simulink model "mwrc04_fullvehicle"  (Simulink 6.0)
settings: Solver=ode3  SolverMode=SingleTasking  StartTime=0.0  StopTime=2  FixedStep=0.001  RelTol=1e-5  AbsTol=1e-6
PreLoadFcn:
  | load fsysdat
undefined symbols (not defined in the file or in its folder): A1, A2, B1, B2, converter_data, DISABLED, downtab, emap, hys, Iei, Ki, LOW, LSB, max_ego, max_press, max_speed, max_throt, min_press, min_throt, Neng_max, o2_t_thresh, Pbar, PressEst, pumpCon, RICH, sigbuilder_block, SpeedEst, ThrotEst, uptab, vehicledata, zero_thresh
libraries: simulink_extras x2, simulink x1
settings Model: Creator=nikita  LastModifiedBy=mshakeri  ExtModeTrigMode=oneshot  ExtModeArmWhenConnect=off  ExtModeAutoUpdateStatusClock=off  ProdHWDeviceType=Specified
settings SolverCC: AutoInsertRateTranBlk=on
settings DataIOCC: LimitDataPoints=off  SignalLoggingName=sigsOut
settings OptimizationCC: MultiInstanced=off
settings FormatCC: IgnoreBidirectionalLines=off
settings DebuggingCC: IntegerOverflowMsg=none
settings HardwareCC: ProdHWDeviceType=Specified
settings RTWCC: SystemTargetFile=ert.tlc  TemplateMakefile=ert_default_tmf  Description=RTW Embedded Coder  ProcessScript=ert_make_rtw_hook
settings CodeAppCC: IgnoreCustomStorageClasses=off  SimulinkBlockComments=off
settings ERTTargetCC: TargetFcnLib=iso_c_tmw.mat  GenerateSampleERTMain=on  GenFloatMathFcnCalls=ANSI_C  RootIOFormat=Individual Arguments  LifeSpan=1  SourceCodeTemplate=example_banner.tlc  HeaderCodeTemplate=example_banner.tlc  SourceDataTemplate=example_banner.tlc  HeaderDataTemplate=example_banner.tlc  ERTCustomFileTemplate=example_file_process.tlc  InitialValueSource=Model

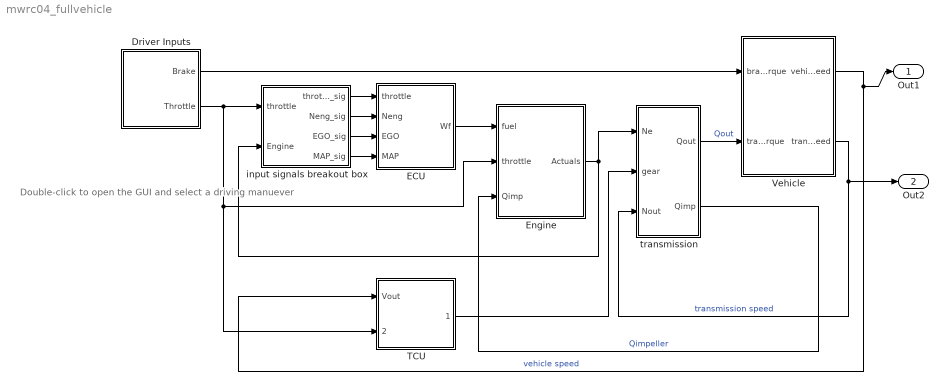
== system mwrc04_fullvehicle ==
  note: Double-click to
      | open the GUI
      | and select a
      | driving manuever
  Driver Inputs : Subsystem  Tag=STV Subsys  StartFcn=sigbuilder_block('start');  StopFcn=sigbuilder_block('stop');  ClipboardFcn=sigbuilder_block('clipboard');  mask(Sigbuilder block){}
      mask help: Sigbuilder GUI
      mask init:
      | tuvar = sigbuilder_block('maskInit');
      settings: CopyFcn=sigbuilder_block('copy');  DeleteFcn=sigbuilder_block('delete');  ModelCloseFcn=sigbuilder_block('modelClose');  PreSaveFcn=sigbuilder_block('preSave');  NameChangeFcn=sigbuilder_block('namechange');  OpenFcn=sigbuilder_block('open',[12 234.75 413.25 257.25 ]);  CloseFcn=sigbuilder_block('close');
      mask Display: plot(0,0,100,100,[10,10,40,40,10],[80,20,20,80,80],[40,10],[50,50], [40,27,10],[65,72,56],[40,25,25,10],[28,28,43,43]);
  ECU : Subsystem  TreatAsAtomicUnit=on
  Engine : Subsystem
  TCU : Subsystem  TreatAsAtomicUnit=on
  Vehicle : Subsystem  mask(vehicle model){Rfd=vehicledata(1), rload0=vehicledata(2), rload2=vehicledata(3), Rw=vehicledata(4), Iv=vehicledata(5), N20=vehicledata(6)/vehicledata(4)*vehicledata(1)}
      mask prompts: Rfd "final drive ratio"; rload0 "drag friction at wheels"; rload2 "aerodynamic drag"; Rw "wheel radius"; Iv "vehicle inertia"; N20 "initial transmission output speed"
      mask help: vehicle dynamics: torque input from trans., outputs are input speed (transmission output) and vehicle speed
      mask Display:
      | port_label('input',1,'Qbrake')
      | port_label('input',2,'Qtrans')
      | port_label('output',1,'Vout')
      | port_label('output',2,'Nout')
  input signals breakout box : Subsystem
  transmission : Subsystem
  Out1 : Outport
  Out2 : Outport  Port=2
  wires:
  ECU/1("Wf ") -> Engine/1(fuel)
  transmission/1(Qout) -> Vehicle/2(transmission output torque)  "Qout"
  Vehicle/1(vehicle speed) -> TCU/1(Vout), Out1/1  "vehicle speed"
  Driver Inputs/1(Brake) -> Vehicle/1(brake torque)
  input signals breakout box/1(throttle_sig) -> ECU/1(throttle)
  input signals breakout box/2(Neng_sig) -> ECU/2(Neng)
  input signals breakout box/3(EGO_sig) -> ECU/3(EGO)
  input signals breakout box/4(MAP_sig) -> ECU/4(MAP)
  TCU/1(gear select) -> transmission/2(gear)
  transmission/2(Qimp) -> Engine/3(Qimp)  "Qimpeller"
  Driver Inputs/2(Throttle) -> Engine/2(throttle), TCU/2(throttle), input signals breakout box/1(throttle)
  Engine/1(Actuals) -> transmission/1(Ne), input signals breakout box/2(Engine)
  Vehicle/2(transmission output speed) -> transmission/3(Nout), Out2/1  "transmission speed"

== system mwrc04_fullvehicle/Driver Inputs ==
  Demux : Demux  Tag=STV Demux  Outputs=2
  FromWs : FromWorkspace  Tag=STV FromWs  VariableName=tuvar  SampleTime=0.001  SigBuilderData=DataTag0
      SigBuilderData=|
      | channels(1).label = 'Brake'
      | channels(1).allXData = {[0 50], [0 50], [0 10 10 50], [0 50]}
      | channels(1).allYData = {[0 0], [0 0], [0 0 325 325], [0 0]}
      | channels(2).label = 'Throttle'
      | channels(2).allXData = {[0 14.9 15 15 50], [0 50], [0 5.1 5.1 50], [0 4.8 4.8 50]}
      | channels(2).allYData = {[60 40 100 100 58.8235294118], [13.4 24], [50 50 1 1], [80 80 1 1]}
      | dataSet(1).timeRange = [0 50]
      | dataSet(1).name = 'Passing Maneuver'
      | dataSet(2).timeRange = [0 50]
      | dataSet(2).name = 'Gradual Acceleration'
      | dataSet(3).timeRange = [0 50]
      | dataSet(3).name = 'Hard braking'
      | dataSet(4).timeRange = [0 50]
      | dataSet(4).name = 'Coasting'
  Brake : Outport  Tag=STV Outport
  Throttle : Outport  Tag=STV Outport  Port=2
  wires:
  FromWs/1 -> Demux/1
  Demux/1 -> Brake/1
  Demux/2 -> Throttle/1

== system mwrc04_fullvehicle/ECU ==
  note: Fuel Rate Control
  note: Physical Inputs
  note: Physical Outputs
  throttle : Inport
  Neng : Inport  Port=2
  EGO : Inport  Port=3
  MAP : Inport  Port=4
  Analog conditioning and conversion : Subsystem
  Analog output conversion : Subsystem
  ECU Application Software : Subsystem  TreatAsAtomicUnit=on
  "Wf " : Outport  InitialOutput=0
  wires:
  ECU Application Software/1(cmdOut) -> Analog output conversion/1(cmdOut)
  throttle/1 -> Analog conditioning and conversion/1(throttle_sig)  "throttle"
  Neng/1 -> Analog conditioning and conversion/2(Neng_sig)  "Neng"
  EGO/1 -> Analog conditioning and conversion/3(EGO_sig)  "EGO"
  MAP/1 -> Analog conditioning and conversion/4(MAP_sig)  "MAP"
  Analog conditioning and conversion/1(senseRaw) -> ECU Application Software/1(senseIn)
  Analog output conversion/1(Wf) -> "Wf "/1

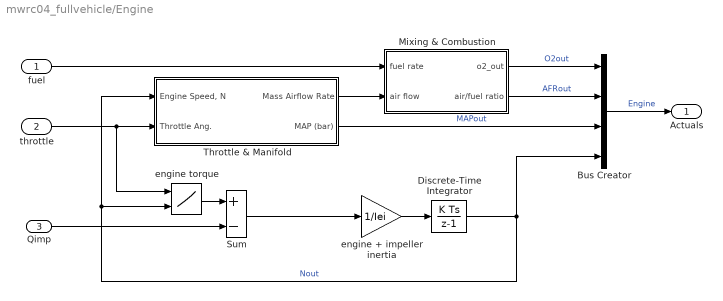
== system mwrc04_fullvehicle/Engine ==
  fuel : Inport
  throttle : Inport  Port=2
  Qimp : Inport  Port=3
  Bus Creator : BusCreator
  Discrete-Time Integrator : DiscreteIntegrator  InitialCondition=1000  LimitOutput=on  UpperSaturationLimit=Neng_max  LowerSaturationLimit=600  SampleTime=0.001
  Mixing & Combustion : Subsystem
  Sum : Sum  Inputs=+-  SaturateOnIntegerOverflow=on  InputSameDT=on
  Throttle & Manifold : Subsystem
  engine torque : Lookup2D  RowIndex=thvec  ColumnIndex=nevec  OutputValues=emap  OutScaling=2^-10  InputSameDT=on
  engine + impeller inertia : Gain  Gain=1/Iei  SaturateOnIntegerOverflow=on
  Actuals : Outport
  wires:
  Throttle & Manifold/1(Mass Airflow Rate) -> Mixing & Combustion/2(air flow)
  fuel/1 -> Mixing & Combustion/1(fuel rate)
  throttle/1 -> Throttle & Manifold/2(Throttle Ang.), engine torque/1
  Mixing & Combustion/2(air/fuel ratio) -> Bus Creator/2  "AFRout"
  Throttle & Manifold/2(MAP (bar)) -> Bus Creator/3  "MAPout"
  Mixing & Combustion/1(o2_out) -> Bus Creator/1  "O2out"
  Bus Creator/1 -> Actuals/1  "Engine"
  Discrete-Time Integrator/1 -> engine torque/2, Throttle & Manifold/1("Engine Speed, N"), Bus Creator/4  "Nout"
  Sum/1 -> engine + impeller inertia/1
  engine + impeller inertia/1 -> Discrete-Time Integrator/1
  engine torque/1 -> Sum/1
  Qimp/1 -> Sum/2

== system mwrc04_fullvehicle/TCU ==
  note: Electronic Shift Control
  Vout : Inport
  throttle : Inport  Port=2
  Threshold Calculation : Subsystem  Orientation=left  TreatAsAtomicUnit=on
  shift_logic : Stateflow chart
  gear select : Outport
  wires:
  Threshold Calculation/1(down_th) -> shift_logic/3(down_th)
  Threshold Calculation/2(up_th) -> shift_logic/2(up_th)
  shift_logic/1(gear) -> Threshold Calculation/1(gear), gear select/1
  shift_logic/2(CALC_TH) -> Threshold Calculation/Trigger
  throttle/1 -> Threshold Calculation/2(throttle)
  Vout/1 -> shift_logic/1(speed)

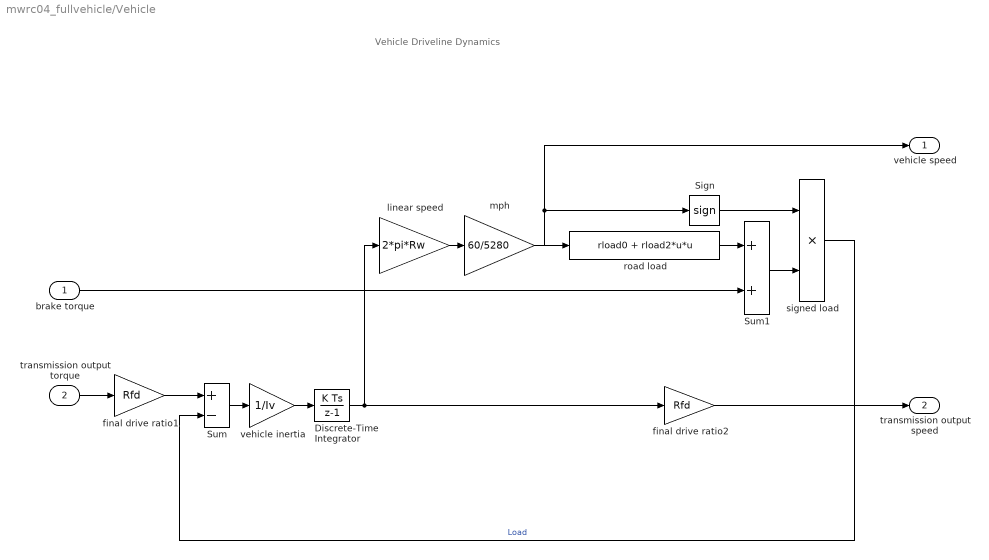
== system mwrc04_fullvehicle/Vehicle ==
  note: Vehicle Driveline Dynamics
  brake torque : Inport
  transmission output torque : Inport  Port=2
  Discrete-Time Integrator : DiscreteIntegrator  InitialCondition=N20/Rfd  SampleTime=0.001
  Sign : Signum
  Sum : Sum  Inputs=+-  SaturateOnIntegerOverflow=on  InputSameDT=on
  Sum1 : Sum  SaturateOnIntegerOverflow=on  InputSameDT=on
  final drive ratio1 : Gain  Gain=Rfd  SaturateOnIntegerOverflow=on
  final drive ratio2 : Gain  Gain=Rfd  SaturateOnIntegerOverflow=on
  linear speed : Gain  Gain=2*pi*Rw  SaturateOnIntegerOverflow=on
  mph : Gain  Gain=60/5280  SaturateOnIntegerOverflow=on
  road load : Fcn  Expr=rload0 + rload2*u*u
  signed load : Product  SaturateOnIntegerOverflow=on  InputSameDT=on
  vehicle inertia : Gain  Gain=1/Iv  SaturateOnIntegerOverflow=on
  vehicle speed : Outport  InitialOutput=0
  transmission output speed : Outport  Port=2  InitialOutput=0
  wires:
  final drive ratio2/1 -> transmission output speed/1
  brake torque/1 -> Sum1/2
  Sum1/1 -> signed load/2
  road load/1 -> Sum1/1
  Sign/1 -> signed load/1
  signed load/1 -> Sum/2  "Load"
  transmission output torque/1 -> final drive ratio1/1
  vehicle inertia/1 -> Discrete-Time Integrator/1
  Sum/1 -> vehicle inertia/1
  mph/1 -> vehicle speed/1, Sign/1, road load/1
  linear speed/1 -> mph/1
  Discrete-Time Integrator/1 -> final drive ratio2/1, linear speed/1
  final drive ratio1/1 -> Sum/1

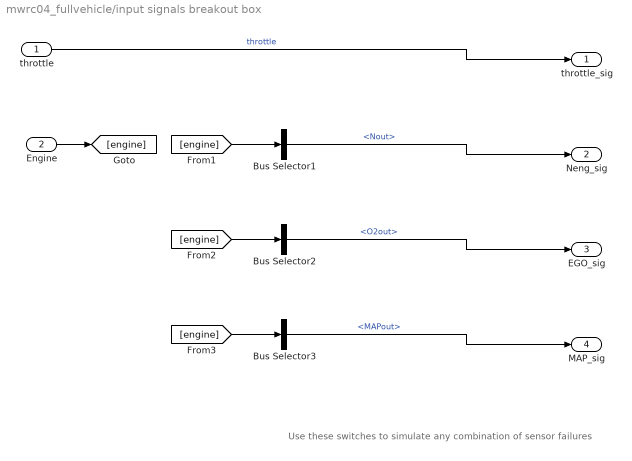
== system mwrc04_fullvehicle/input signals breakout box ==
  note: Use these switches to
      | simulate any combination
      | of sensor failures
  throttle : Inport
  Engine : Inport  Port=2
  Bus Selector1 : BusSelector  OutputSignals=Nout
  Bus Selector2 : BusSelector  OutputSignals=O2out
  Bus Selector3 : BusSelector  OutputSignals=MAPout
  throttle_sig : Outport
  Neng_sig : Outport  Port=2
  EGO_sig : Outport  Port=3
  MAP_sig : Outport  Port=4
  wires:
  throttle/1 -> throttle_sig/1  "throttle"
  Bus Selector2/1 -> EGO_sig/1  "<O2out>"
  Bus Selector3/1 -> MAP_sig/1  "<MAPout>"
  Bus Selector1/1 -> Neng_sig/1  "<Nout>"
  Engine/1 -> [engine]
  [engine] -> Bus Selector1/1
  [engine] -> Bus Selector2/1
  [engine] -> Bus Selector3/1

== system mwrc04_fullvehicle/transmission ==
  Ne : Inport
  gear : Inport  Port=2
  Nout : Inport  Port=3
  Bus Selector1 : BusSelector  OutputSignals=Nout
  Torque Converter : Subsystem  mask(torque converter){speedratio=converter_data(:,1), Kfactor=converter_data(:,2), Torkratio=converter_data(:,3)}
      mask prompts: speedratio "speed ratio"; Kfactor "K factor"; Torkratio "torque ratio"
      mask help: torque converter
      mask Help: Torque converter input and output torques are computed as a function of the input and output speeds
      mask Display: plot([cos([90:10:450]*pi/180),.63*cos([90:10:450]*pi/180),.63*cos([90:10:240]*pi/180),cos([240:10:300]*pi/180),.63*cos([300]*pi/180)],[sin([90:10:450]*pi/180),.63*sin([90:10:450]*pi/180)+.1,.63*sin([90:10:240]*pi/180)+.1,sin([240:10:300]*pi/180),.63*sin([300]*pi/180)+.1])
  transmission ratio : Subsystem
  Qout : Outport  InitialOutput=0
  Qimp : Outport  Port=2  InitialOutput=0
  wires:
  transmission ratio/1(Tout) -> Qout/1
  Torque Converter/1(Ti) -> Qimp/1
  Nout/1 -> transmission ratio/3(Nout)
  gear/1 -> transmission ratio/2(gear)
  Ne/1 -> Bus Selector1/1
  transmission ratio/2(Nin) -> Torque Converter/2(Nin)
  Torque Converter/2(Tt) -> transmission ratio/1(Tin)  "turbine torque"
  Bus Selector1/1 -> Torque Converter/1(Neng)  "<Nout>"

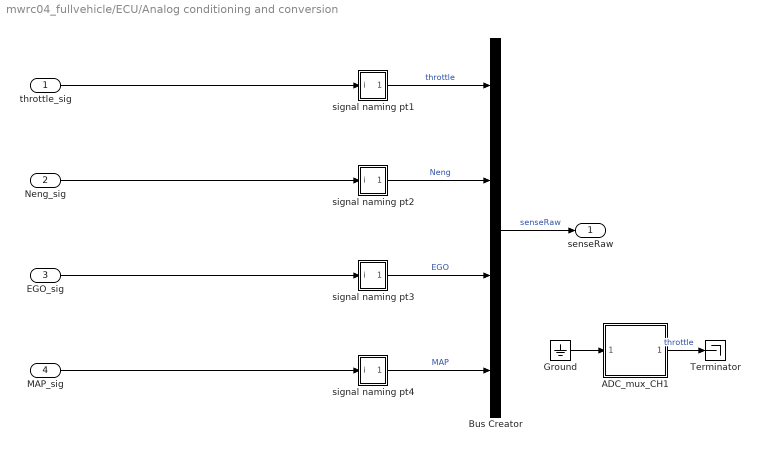
== system mwrc04_fullvehicle/ECU/Analog conditioning and conversion ==
  throttle_sig : Inport
  Neng_sig : Inport  Port=2
  EGO_sig : Inport  Port=3
  MAP_sig : Inport  Port=4
  ADC_mux_CH1 : Subsystem  mask(IdealADC){NumberOfConverterBits=8, Vmin=0, Vmax=5, OutputDataType=double}
      mask prompts: NumberOfConverterBits "Number of converter bits:"; Vmin "Min input voltage at low output:"; Vmax "Max input voltage at 2^n output (unreachable):"; OutputDataType "Output data type:"
      mask help: Idealized analog to digital converter. There are 2^n possible digital output codes for an n-bit converter. Each value represents an equal fraction of the total analog input range in steps of one least significant bit (1 LSB). 1 LSB is (Vmax - Vmin)/2^bits. The midpoint of these steps corresponds to the actual value and thus introduce quantization error that is never more than 1/2 LSB. Since the first and last steps in the converter's range are only 1/2 LSB in width, the full scale range (FSR) of the converter is equal to (2^n - 1) step widths. The FSR low transition occurs at Vmin + 1/2 LSB, the FSR high transition occurs at Vmax - 3/2 LSB. When the block output is a floating point type, int32 is used for truncation. Conversion time is zero in this model.
      mask init:
      | [LSB,steps_x,steps_y,line_xy] = sl_addamask(NumberOfConverterBits,Vmin,Vmax,OutputDataType);
      settings: AttributesFormatString=(settings: %<NumberOfConverterBits>-bit converter\nVmin: %<Vmin>, Vmax: %<Vmax>)
      mask Help: Use this block to model an ideal analog to digital converter.  To model non-ideal converters, it is suggested to use a direct look-up table to represent static errors and dynamic models for transient error sources.  Use a discrete delay of the appropriate duration to model conversion latency if this is a significant value in your application.  If there is an input mux, model this with triggered latencies on the input side of the A/D block.
      mask StyleString: edit,edit,edit,popup(double|single|int8|uint8|int16|uint16|int32|uint32|boolean)
      mask Display:
      | plot(steps_x,steps_y)
      | plot(line_xy, line_xy)
      | port_label('input',1,'A')
      | port_label('output',1,'D')
      | text(0.5,0.9,[num2str(NumberOfConverterBits),' bits'],'horizontalalignment','center')
  Bus Creator : BusCreator
  Ground : Ground
  Terminator : Terminator
  signal naming pt1 : Subsystem
  signal naming pt2 : Subsystem
  signal naming pt3 : Subsystem
  signal naming pt4 : Subsystem
  senseRaw : Outport
  wires:
  Bus Creator/1 -> senseRaw/1  "senseRaw"
  throttle_sig/1 -> signal naming pt1/1(i)
  Neng_sig/1 -> signal naming pt2/1(i)
  EGO_sig/1 -> signal naming pt3/1(i)
  MAP_sig/1 -> signal naming pt4/1(i)
  signal naming pt1/1(o) -> Bus Creator/1  "throttle"
  signal naming pt2/1(o) -> Bus Creator/2  "Neng"
  signal naming pt3/1(o) -> Bus Creator/3  "EGO"
  signal naming pt4/1(o) -> Bus Creator/4  "MAP"
  ADC_mux_CH1/1(Digital Counts) -> Terminator/1  "throttle"
  Ground/1 -> ADC_mux_CH1/1(Sampled Volts)

== system mwrc04_fullvehicle/ECU/Analog output conversion ==
  cmdOut : Inport
  Bus Selector : BusSelector  OutputSignals=Wfcmd
  signal naming pt1 : Subsystem
  Wf : Outport
  wires:
  cmdOut/1 -> Bus Selector/1
  Bus Selector/1 -> signal naming pt1/1(i)  "<Wfcmd>"
  signal naming pt1/1(o) -> Wf/1  "Wf"

== system mwrc04_fullvehicle/ECU/ECU Application Software ==
  note: ECU Application - Top Level
  senseIn : Inport
  Airflow calculation : Subsystem  TreatAsAtomicUnit=on
  Fuel  Calculation : Subsystem  TreatAsAtomicUnit=on
  Input Signal Conversion : Subsystem  TreatAsAtomicUnit=on
  Mode Logic : Subsystem  TreatAsAtomicUnit=on
  Output Signal Conversion : Subsystem  TreatAsAtomicUnit=on
  Sensor correction and  Fault Redundancy : Subsystem  TreatAsAtomicUnit=on
  cmdOut : Outport
  wires:
  Mode Logic/2(fuel_mode) -> Fuel  Calculation/4(mode), Airflow calculation/3(mode)
  Airflow calculation/2(feedback correction) -> Fuel  Calculation/2(feedback correction)
  Airflow calculation/1(est. air flow) -> Fuel  Calculation/1(est. air flow)
  Sensor correction and  Fault Redundancy/1(corrected) -> Airflow calculation/1(sens_in)
  Mode Logic/1(fail_state) -> Sensor correction and  Fault Redundancy/2(failures), Airflow calculation/2(Failures), Fuel  Calculation/3(Failures)
  senseIn/1 -> Input Signal Conversion/1(senseRaw)
  Fuel  Calculation/1(Cmd) -> Output Signal Conversion/1(Cmd)
  Output Signal Conversion/1(cmdOut) -> cmdOut/1
  Input Signal Conversion/1(sensors) -> Sensor correction and  Fault Redundancy/1(sensors), Mode Logic/1(sensors)

== system mwrc04_fullvehicle/Engine/Mixing & Combustion ==
  fuel rate : Inport
  air flow : Inport  Port=2
  Constant4 : Constant  Orientation=up  Value=0.1
  Discrete Transfer Fcn : DiscreteTransferFcn  Numerator=3  Denominator=[1 3]  SampleTime=0.001
  EGO Sensor : Fcn  Expr=(1-tanh(4*(u[1]-14.6)))/2
  MinMax : MinMax  Function=max  Inputs=2  SaturateOnIntegerOverflow=on  InputSameDT=on
  Product : Product  Inputs=*/  SaturateOnIntegerOverflow=on  InputSameDT=on
  o2_out : Outport  InitialOutput=0
  air/fuel ratio : Outport  Port=2  InitialOutput=0
  wires:
  Constant4/1 -> MinMax/2
  fuel rate/1 -> MinMax/1
  MinMax/1 -> Product/2
  Product/1 -> Discrete Transfer Fcn/1
  Discrete Transfer Fcn/1 -> air/fuel ratio/1, EGO Sensor/1
  EGO Sensor/1 -> o2_out/1
  air flow/1 -> Product/1

== system mwrc04_fullvehicle/Engine/Throttle & Manifold ==
  note: Air-Fuel Intake Dynamics
  "Engine Speed, N" : Inport
  Throttle Ang. : Inport  Port=2
  "Atmospheric Pressure, Pa (bar)" : Constant  Value=Pbar
  Intake Manifold : Subsystem
  Limit to Positive : Saturate  UpperLimit=inf  LowerLimit=0
  Throttle : Subsystem
  Mass Airflow Rate : Outport  InitialOutput=0
  MAP (bar) : Outport  Port=2  InitialOutput=0
  wires:
  Limit to Positive/1 -> Throttle/1("Throttle Angle, theta (deg)")
  Throttle Ang./1 -> Limit to Positive/1
  Throttle/1("Throttle  Flow, mdot  (g/s)") -> Intake Manifold/1(mdot Input  (g/s))
  "Engine Speed, N"/1 -> Intake Manifold/2(N (rad/sec))
  Intake Manifold/1(mdot to Cylinder  (g/s)) -> Mass Airflow Rate/1
  "Atmospheric Pressure, Pa (bar)"/1 -> Throttle/3("Atmospheric Pressure, Pa (bar) ")
  Intake Manifold/2("Manifold Pressure, Pm (bar)") -> Throttle/2("Manifold Pressure, Pm (bar)"), MAP (bar)/1

== system mwrc04_fullvehicle/TCU/Threshold Calculation ==
  gear : Inport
  throttle : Inport  Port=2
  run : TriggerPort  TriggerType=function-call  ZeroCross=off
  interp_down : Lookup2D  RowIndex=downth  ColumnIndex=[1:4]  OutputValues=downtab  OutScaling=2^-10  InputSameDT=on
  interp_up : Lookup2D  RowIndex=upth  ColumnIndex=[1:4]  OutputValues=uptab  OutScaling=2^-10  InputSameDT=on
  down_th : Outport
  up_th : Outport  Port=2
  wires:
  interp_up/1 -> up_th/1
  interp_down/1 -> down_th/1
  throttle/1 -> interp_up/1, interp_down/1
  gear/1 -> interp_up/2, interp_down/2

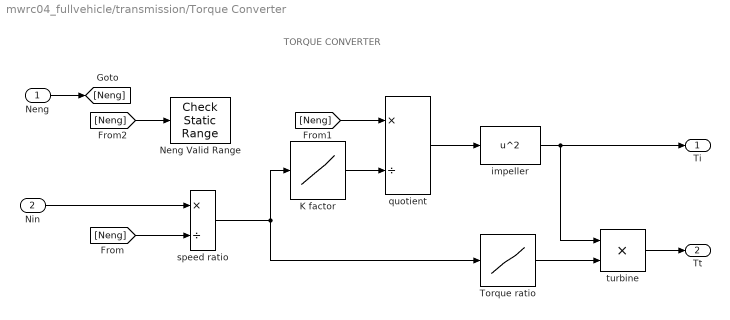
== system mwrc04_fullvehicle/transmission/Torque Converter ==
  note: TORQUE CONVERTER
  Neng : Inport
  Nin : Inport  Port=2
  K factor : Lookup  InputValues=speedratio  OutputValues=Kfactor  SaturateOnIntegerOverflow=on
  Neng Valid Range : simulink/Model Verification/Check  Static Range  Description=0 < u <= Neng_max  max=Neng_max  max_included=on  min=0  min_included=off  enabled=on  stopWhenAssertionFail=on  export=off  icon=graphic
      settings: AttributesFormatString=%<min> <= u <= %<max>
  Torque ratio : Lookup  InputValues=speedratio  OutputValues=Torkratio  SaturateOnIntegerOverflow=on
  impeller : Fcn  Expr=u^2
  quotient : Product  Inputs=*/  SaturateOnIntegerOverflow=on  InputSameDT=on
  speed ratio : Product  Inputs=*/  SaturateOnIntegerOverflow=on  InputSameDT=on
  turbine : Product  SaturateOnIntegerOverflow=on  InputSameDT=on
  Ti : Outport  InitialOutput=0
  Tt : Outport  Port=2  InitialOutput=0
  wires:
  quotient/1 -> impeller/1
  K factor/1 -> quotient/2
  impeller/1 -> Ti/1, turbine/1
  turbine/1 -> Tt/1
  Nin/1 -> speed ratio/1
  Torque ratio/1 -> turbine/2
  [Neng] -> speed ratio/2
  Neng/1 -> [Neng]
  [Neng] -> quotient/1
  [Neng] -> Neng Valid Range/1
  speed ratio/1 -> K factor/1, Torque ratio/1

== system mwrc04_fullvehicle/transmission/transmission ratio ==
  Tin : Inport
  gear : Inport  Port=2
  Nout : Inport  Orientation=left  Port=3
  Look-Up Table : Lookup  InputValues=[1 2 3 4]  OutputValues=[2.393 1.450 1.000 0.677]  SaturateOnIntegerOverflow=on
  Product : Product  SaturateOnIntegerOverflow=on  InputSameDT=on
  Product1 : Product  Orientation=left  SaturateOnIntegerOverflow=on  InputSameDT=on
  Tout : Outport  InitialOutput=0
  Nin : Outport  Orientation=left  Port=2  InitialOutput=0
  wires:
  Look-Up Table/1 -> Product1/1, Product/2
  Nout/1 -> Product1/2
  Product1/1 -> Nin/1
  Product/1 -> Tout/1
  Tin/1 -> Product/1
  gear/1 -> Look-Up Table/1

== system mwrc04_fullvehicle/ECU/Analog conditioning and conversion/ADC_mux_CH1 ==
  Sampled Volts : Inport
  ADC Counts Range divided by Input Voltage Range : Gain  Gain=1/LSB  SaturateOnIntegerOverflow=on
  Cause rounding behavior upon truncation : Constant  Orientation=up  Value=0.5
  Saturate voltage  to output range : Saturate  UpperLimit=Vmax - 1.5 * LSB  LowerLimit=Vmin + 0.5 * LSB
      settings: AttributesFormatString=Max = %<UpperLimit>\nMin = %<LowerLimit>
  Sum : Sum  Inputs=|++  SaturateOnIntegerOverflow=on
  cast : DataTypeConversion  OutDataTypeMode=double  RndMeth=Zero
  truncate : DataTypeConversion  OutDataTypeMode=int32  SaturateOnIntegerOverflow=on  RndMeth=Zero
  Digital Counts : Outport
  wires:
  Sampled Volts/1 -> Saturate voltage  to output range/1
  truncate/1 -> cast/1
  ADC Counts Range divided by Input Voltage Range/1 -> Sum/1
  Sum/1 -> truncate/1
  Cause rounding behavior upon truncation/1 -> Sum/2
  Saturate voltage  to output range/1 -> ADC Counts Range divided by Input Voltage Range/1
  cast/1 -> Digital Counts/1

== system mwrc04_fullvehicle/ECU/Analog conditioning and conversion/signal naming pt1 ==
  i : Inport
  o : Outport
  wires:
  i/1 -> o/1

== system mwrc04_fullvehicle/ECU/Analog conditioning and conversion/signal naming pt2 ==
  i : Inport
  o : Outport
  wires:
  i/1 -> o/1

== system mwrc04_fullvehicle/ECU/Analog conditioning and conversion/signal naming pt3 ==
  i : Inport
  o : Outport
  wires:
  i/1 -> o/1

== system mwrc04_fullvehicle/ECU/Analog conditioning and conversion/signal naming pt4 ==
  i : Inport
  o : Outport
  wires:
  i/1 -> o/1

== system mwrc04_fullvehicle/ECU/Analog output conversion/signal naming pt1 ==
  i : Inport
  o : Outport
  wires:
  i/1 -> o/1

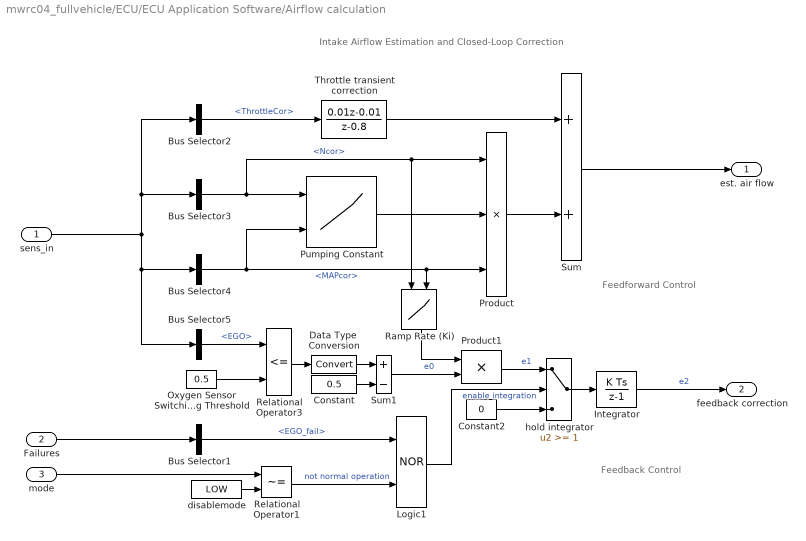
== system mwrc04_fullvehicle/ECU/ECU Application Software/Airflow calculation ==
  note: Intake Airflow Estimation and Closed-Loop Correction
  note: Feedback Control
  note: Feedforward Control
  sens_in : Inport
  Failures : Inport  Port=2
  mode : Inport  Port=3
  Bus Selector1 : BusSelector  OutputSignals=EGO_fail
  Bus Selector2 : BusSelector  OutputSignals=ThrottleCor
  Bus Selector3 : BusSelector  OutputSignals=Ncor
  Bus Selector4 : BusSelector  OutputSignals=MAPcor
  Bus Selector5 : BusSelector  OutputSignals=EGO
  Constant : Constant  Value=0.5
  Constant2 : Constant  Value=0
  Data Type  Conversion : DataTypeConversion  OutDataTypeMode=double  SaturateOnIntegerOverflow=on  RndMeth=Zero
  Integrator : DiscreteIntegrator  InitialCondition=-0.01  SampleTime=.01
  Logic1 : Logic  Operator=NOR
  Oxygen Sensor Switching Threshold : Constant  Value=0.5
  Product : Product  Inputs=3  SaturateOnIntegerOverflow=on  InputSameDT=on
  Product1 : Product  SaturateOnIntegerOverflow=on  InputSameDT=on
  Pumping Constant : Lookup2D  RowIndex=SpeedVect  ColumnIndex=press  OutputValues=pumpCon  SaturateOnIntegerOverflow=on  InputSameDT=on
  Ramp Rate (Ki) : Lookup2D  Orientation=down  RowIndex=[100:100:500]  ColumnIndex=[0:0.2:1]  OutputValues=[1:5]'*[1:6]*Ki  SaturateOnIntegerOverflow=on  InputSameDT=on
  Relational Operator1 : RelationalOperator  Operator=~=  InputSameDT=on
  Relational Operator3 : RelationalOperator  Operator=<=  InputSameDT=on
  Sum : Sum  Inputs=2  SaturateOnIntegerOverflow=on  InputSameDT=on
  Sum1 : Sum  Inputs=+-  SaturateOnIntegerOverflow=on  InputSameDT=on
  Throttle transient correction : DiscreteTransferFcn  Numerator=[0.01 -0.01]  Denominator=[1 -0.8]  SampleTime=.01
  disablemode : Constant  Value=LOW
  hold integrator : Switch  Threshold=1  SaturateOnIntegerOverflow=on  InputSameDT=on
  est. air flow : Outport  InitialOutput=0
  feedback correction : Outport  Port=2  InitialOutput=0
  wires:
  Integrator/1 -> feedback correction/1  "e2"
  mode/1 -> Relational Operator1/1
  sens_in/1 -> Bus Selector5/1, Bus Selector4/1, Bus Selector2/1, Bus Selector3/1
  Pumping Constant/1 -> Product/2
  Product/1 -> Sum/2
  Bus Selector4/1 -> Ramp Rate (Ki)/2, Product/3, Pumping Constant/2  "<MAPcor>"
  Bus Selector3/1 -> Pumping Constant/1, Product/1, Ramp Rate (Ki)/1  "<Ncor>"
  Throttle transient correction/1 -> Sum/1
  Sum/1 -> est. air flow/1
  Bus Selector2/1 -> Throttle transient correction/1  "<ThrottleCor>"
  Bus Selector1/1 -> Logic1/1  "<EGO_fail>"
  Failures/1 -> Bus Selector1/1
  disablemode/1 -> Relational Operator1/2
  Relational Operator1/1 -> Logic1/2  "not normal operation"
  Bus Selector5/1 -> Relational Operator3/1  "<EGO>"
  Oxygen Sensor Switching Threshold/1 -> Relational Operator3/2
  Ramp Rate (Ki)/1 -> Product1/1
  Constant2/1 -> hold integrator/3
  Product1/1 -> hold integrator/1  "e1"
  hold integrator/1 -> Integrator/1
  Logic1/1 -> hold integrator/2  "enable integration"
  Sum1/1 -> Product1/2  "e0"
  Relational Operator3/1 -> Data Type  Conversion/1
  Data Type  Conversion/1 -> Sum1/1
  Constant/1 -> Sum1/2

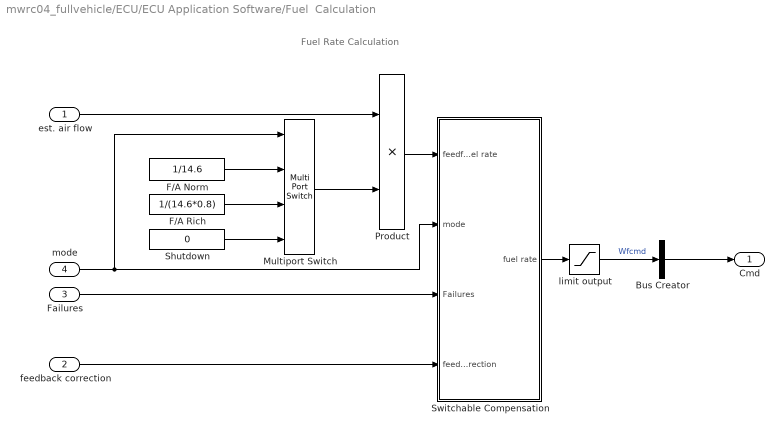
== system mwrc04_fullvehicle/ECU/ECU Application Software/Fuel  Calculation ==
  note: Fuel Rate Calculation
  est. air flow : Inport
  feedback correction : Inport  Port=2
  Failures : Inport  Port=3
  mode : Inport  Port=4
  Bus Creator : BusCreator  Inputs=1
  F/A Norm : Constant  Value=1/14.6
  F/A Rich : Constant  Value=1/(14.6*0.8)
  Multiport Switch : MultiPortSwitch  Inputs=3  SaturateOnIntegerOverflow=on  InputSameDT=on
  Product : Product  SaturateOnIntegerOverflow=on  InputSameDT=on
  Shutdown : Constant  Value=0
  Switchable Compensation : Subsystem
  limit output : Saturate  UpperLimit=100  LowerLimit=0
  Cmd : Outport  InitialOutput=0
  wires:
  limit output/1 -> Bus Creator/1  "Wfcmd"
  feedback correction/1 -> Switchable Compensation/4(feedback correction)
  Shutdown/1 -> Multiport Switch/4
  F/A Rich/1 -> Multiport Switch/3
  F/A Norm/1 -> Multiport Switch/2
  est. air flow/1 -> Product/1
  Multiport Switch/1 -> Product/2
  mode/1 -> Switchable Compensation/2(mode), Multiport Switch/1
  Failures/1 -> Switchable Compensation/3(Failures)
  Product/1 -> Switchable Compensation/1(feedforward fuel rate)
  Switchable Compensation/1(fuel rate) -> limit output/1
  Bus Creator/1 -> Cmd/1

== system mwrc04_fullvehicle/ECU/ECU Application Software/Input Signal Conversion ==
  note: Convert A/D counts to engineering units,
      | accounting for sensor nonlinearities
  senseRaw : Inport
  sensors : Outport
  wires:
  senseRaw/1 -> sensors/1

== system mwrc04_fullvehicle/ECU/ECU Application Software/Mode Logic ==
  sensors : Inport
  Bus Creator : BusCreator
  Bus Selector : BusSelector  OutputSignals=throttle,Neng,EGO,MAP
  Demux : Demux
  control logic : Stateflow chart  Description=Stateflow diagram to determine control system operating mode
  fail_state : Outport
  fuel_mode : Outport  Port=2
  wires:
  control logic/2(fuel_mode) -> fuel_mode/1
  sensors/1 -> Bus Selector/1
  Bus Selector/1 -> control logic/1(throt)  "<throttle>"
  Bus Selector/2 -> control logic/2(speed)  "<Neng>"
  Bus Selector/3 -> control logic/3(Ego)  "<EGO>"
  Bus Selector/4 -> control logic/4(press)  "<MAP>"
  control logic/1(fail_state) -> Demux/1
  Demux/1 -> Bus Creator/1  "throttle_fail"
  Demux/2 -> Bus Creator/2  "Neng_fail"
  Demux/3 -> Bus Creator/3  "EGO_fail"
  Demux/4 -> Bus Creator/4  "MAP_fail"
  Bus Creator/1 -> fail_state/1

== system mwrc04_fullvehicle/ECU/ECU Application Software/Output Signal Conversion ==
  note: Convert engineering units to D/A counts,
      | accounting for output nonlinearities
  Cmd : Inport
  cmdOut : Outport
  wires:
  Cmd/1 -> cmdOut/1

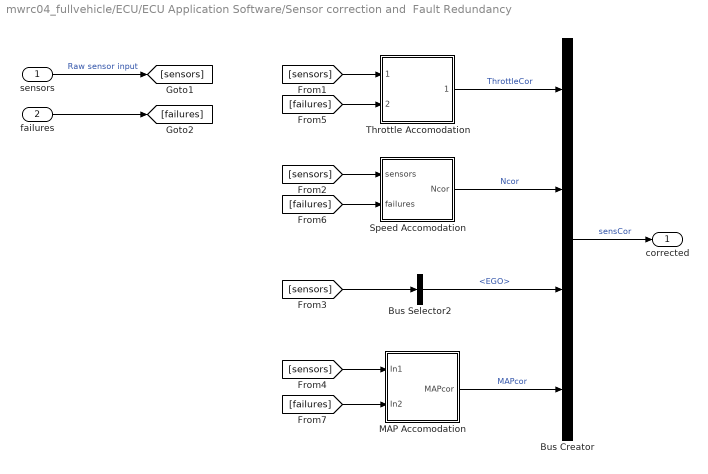
== system mwrc04_fullvehicle/ECU/ECU Application Software/Sensor correction and  Fault Redundancy ==
  sensors : Inport
  failures : Inport  Port=2
  Bus Creator : BusCreator
  Bus Selector2 : BusSelector  OutputSignals=EGO
  MAP Accomodation : Subsystem
  Speed Accomodation : Subsystem
  Throttle Accomodation : Subsystem
  corrected : Outport  InitialOutput=0
  wires:
  MAP Accomodation/1(MAPcor) -> Bus Creator/4  "MAPcor"
  Speed Accomodation/1(Ncor) -> Bus Creator/2  "Ncor"
  Throttle Accomodation/1(ThrottleCor) -> Bus Creator/1  "ThrottleCor"
  Bus Creator/1 -> corrected/1  "sensCor"
  Bus Selector2/1 -> Bus Creator/3  "<EGO>"
  sensors/1 -> [sensors]  "Raw sensor input"
  [sensors] -> Throttle Accomodation/1(sensors)
  [sensors] -> Speed Accomodation/1(sensors)
  [sensors] -> Bus Selector2/1
  [sensors] -> MAP Accomodation/1(In1)
  failures/1 -> [failures]
  [failures] -> Throttle Accomodation/2(failures)
  [failures] -> Speed Accomodation/2(failures)
  [failures] -> MAP Accomodation/2(In2)

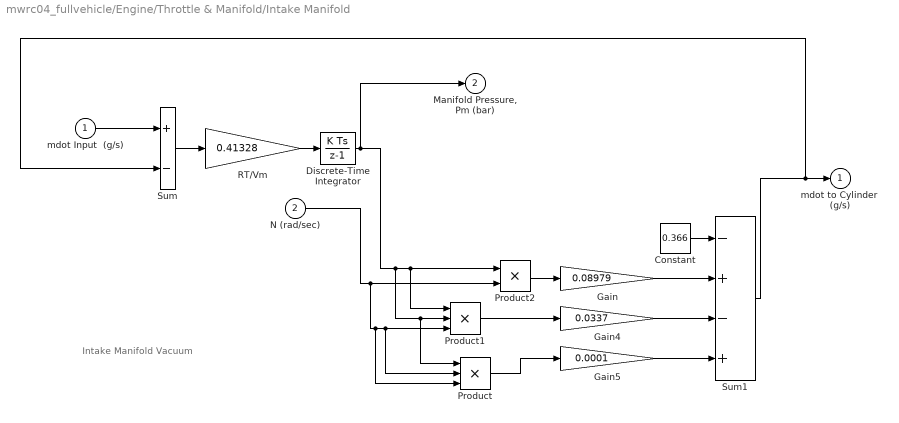
== system mwrc04_fullvehicle/Engine/Throttle & Manifold/Intake Manifold ==
  note: Intake Manifold Vacuum
  mdot Input  (g/s) : Inport
  N (rad/sec) : Inport  Port=2
  Constant : Constant  Value=0.366
  Discrete-Time Integrator : DiscreteIntegrator  InitialCondition=0.589  SampleTime=0.001
  Gain : Gain  Gain=0.08979
  Gain4 : Gain  Gain=0.0337
  Gain5 : Gain  Gain=0.0001
  Product : Product  Inputs=3  RndMeth=Zero
  Product1 : Product  Inputs=3  RndMeth=Zero
  Product2 : Product  RndMeth=Zero
  RT/Vm : Gain  Gain=0.41328  SaturateOnIntegerOverflow=on
  Sum : Sum  Inputs=+-  SaturateOnIntegerOverflow=on  InputSameDT=on
  Sum1 : Sum  Inputs=-+-+
  mdot to Cylinder  (g/s) : Outport  InitialOutput=0
  "Manifold Pressure, Pm (bar)" : Outport  Port=2  InitialOutput=0
  wires:
  mdot Input  (g/s)/1 -> Sum/1
  RT/Vm/1 -> Discrete-Time Integrator/1
  N (rad/sec)/1 -> Product2/2, Product1/3, Product/2, Product/3
  Discrete-Time Integrator/1 -> "Manifold Pressure, Pm (bar)"/1, Product2/1, Product1/1, Product1/2, Product/1
  Sum/1 -> RT/Vm/1
  Sum1/1 -> Sum/2, mdot to Cylinder  (g/s)/1
  Constant/1 -> Sum1/1
  Gain/1 -> Sum1/2
  Gain4/1 -> Sum1/3
  Gain5/1 -> Sum1/4
  Product2/1 -> Gain/1
  Product1/1 -> Gain4/1
  Product/1 -> Gain5/1

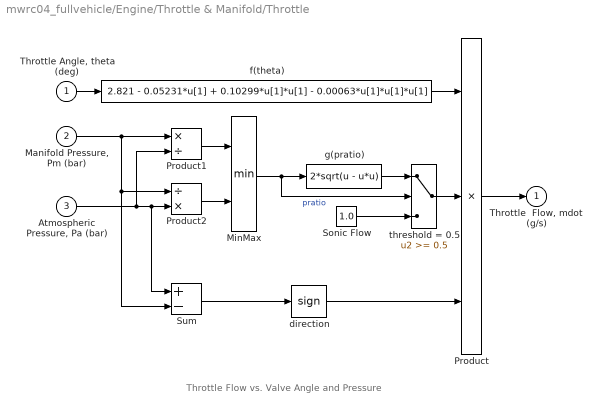
== system mwrc04_fullvehicle/Engine/Throttle & Manifold/Throttle ==
  note: Throttle Flow vs. Valve Angle and Pressure
  "Throttle Angle, theta (deg)" : Inport
  "Manifold Pressure, Pm (bar)" : Inport  Port=2
  "Atmospheric Pressure, Pa (bar) " : Inport  Port=3
  MinMax : MinMax  Inputs=2  SaturateOnIntegerOverflow=on  InputSameDT=on
  Product : Product  Inputs=3  SaturateOnIntegerOverflow=on  InputSameDT=on
  Product1 : Product  Inputs=*/  SaturateOnIntegerOverflow=on  InputSameDT=on
  Product2 : Product  Inputs=/*  SaturateOnIntegerOverflow=on  InputSameDT=on
  "Sonic Flow " : Constant  Value=1.0
  Sum : Sum  Inputs=+-  SaturateOnIntegerOverflow=on  InputSameDT=on
  direction : Signum
  f(theta) : Fcn  Expr=2.821 - 0.05231*u[1] + 0.10299*u[1]*u[1] - 0.00063*u[1]*u[1]*u[1]
  g(pratio) : Fcn  Expr=2*sqrt(u - u*u)
  threshold = 0.5 : Switch  Threshold=0.5  SaturateOnIntegerOverflow=on  InputSameDT=on
  "Throttle  Flow, mdot  (g/s)" : Outport  InitialOutput=0
  wires:
  "Manifold Pressure, Pm (bar)"/1 -> Sum/2, Product2/1, Product1/1
  Product2/1 -> MinMax/2
  Product1/1 -> MinMax/1
  "Atmospheric Pressure, Pa (bar) "/1 -> Sum/1, Product2/2, Product1/2
  g(pratio)/1 -> threshold = 0.5/1
  "Sonic Flow "/1 -> threshold = 0.5/3
  threshold = 0.5/1 -> Product/2
  direction/1 -> Product/3
  Sum/1 -> direction/1
  MinMax/1 -> threshold = 0.5/2, g(pratio)/1  "pratio"
  "Throttle Angle, theta (deg)"/1 -> f(theta)/1
  Product/1 -> "Throttle  Flow, mdot  (g/s)"/1
  f(theta)/1 -> Product/1

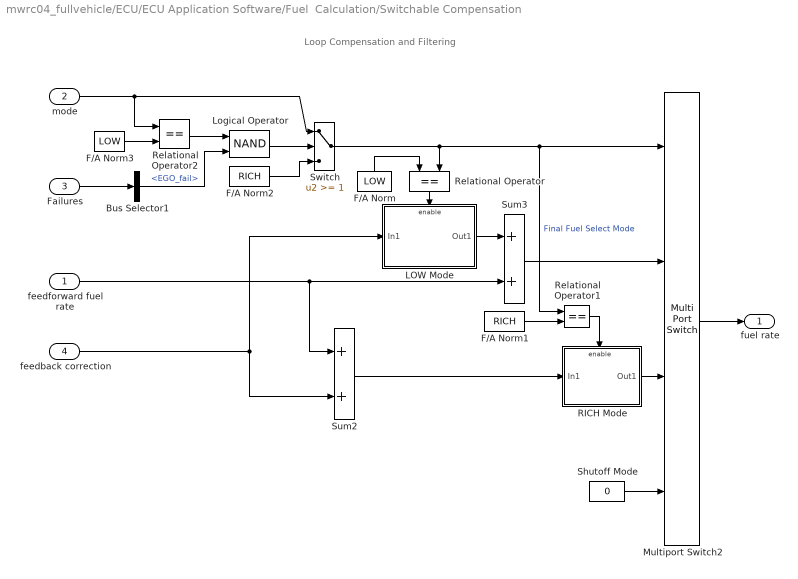
== system mwrc04_fullvehicle/ECU/ECU Application Software/Fuel  Calculation/Switchable Compensation ==
  note: Loop Compensation and Filtering
  feedforward fuel rate : Inport
  mode : Inport  Port=2
  Failures : Inport  Port=3
  feedback correction : Inport  Port=4
  Bus Selector1 : BusSelector  OutputSignals=EGO_fail
  F/A Norm : Constant  Orientation=up  Value=LOW
  F/A Norm1 : Constant  Value=RICH
  F/A Norm2 : Constant  Value=RICH
  F/A Norm3 : Constant  Value=LOW
  LOW Mode : Subsystem  mask(enabled discrete-time transfer function){num=B1, den=A1, u0=-0.01, y0=-0.01, Ts=0.01}
      mask prompts: num "numerator polynomial"; den "denominator polynomial"; u0 "initial input"; y0 "initial output"; Ts "sample time"
      mask Display: dpoly(num,den,'z')
  Logical Operator : Logic  Operator=NAND
  Multiport Switch2 : MultiPortSwitch  Inputs=3  SaturateOnIntegerOverflow=on  InputSameDT=on
  RICH Mode : Subsystem  mask(enabled discrete-time transfer function){num=B2, den=A2, u0=1.6, y0=1.6, Ts=0.01}
      mask prompts: num "numerator polynomial"; den "denominator polynomial"; u0 "initial input"; y0 "initial output"; Ts "sample time"
      mask Display: dpoly(num,den,'z')
  Relational Operator : RelationalOperator  Orientation=down  Operator===  InputSameDT=on
  Relational Operator1 : RelationalOperator  Operator===  InputSameDT=on
  Relational Operator2 : RelationalOperator  Operator===  InputSameDT=on
  Shutoff Mode : Constant  Value=0
  Sum2 : Sum  SaturateOnIntegerOverflow=on  InputSameDT=on
  Sum3 : Sum  SaturateOnIntegerOverflow=on  InputSameDT=on
  Switch : Switch  Threshold=1  SaturateOnIntegerOverflow=on  InputSameDT=on
  fuel rate : Outport  InitialOutput=0
  wires:
  feedforward fuel rate/1 -> Sum3/2, Sum2/1
  feedback correction/1 -> LOW Mode/1(In1), Sum2/2
  RICH Mode/1(Out1) -> Multiport Switch2/3
  LOW Mode/1(Out1) -> Sum3/1
  Sum3/1 -> Multiport Switch2/2
  Sum2/1 -> RICH Mode/1(In1)
  Shutoff Mode/1 -> Multiport Switch2/4
  F/A Norm1/1 -> Relational Operator1/2
  Relational Operator1/1 -> RICH Mode/Enable
  Relational Operator/1 -> LOW Mode/Enable
  Multiport Switch2/1 -> fuel rate/1
  Switch/1 -> Relational Operator1/1, Multiport Switch2/1, Relational Operator/2  "Final Fuel Select Mode"
  F/A Norm/1 -> Relational Operator/1
  F/A Norm2/1 -> Switch/3
  Logical Operator/1 -> Switch/2
  mode/1 -> Switch/1, Relational Operator2/1
  F/A Norm3/1 -> Relational Operator2/2
  Relational Operator2/1 -> Logical Operator/1
  Failures/1 -> Bus Selector1/1
  Bus Selector1/1 -> Logical Operator/2  "<EGO_fail>"

== system mwrc04_fullvehicle/ECU/ECU Application Software/Sensor correction and  Fault Redundancy/MAP Accomodation ==
  In1 : Inport
  In2 : Inport  Port=2
  Bus Selector1 : BusSelector  OutputSignals=MAP_fail
  Bus Selector2 : BusSelector  OutputSignals=MAP
  MAP Estimate : Subsystem
  Switch4 : Switch  Threshold=1  SaturateOnIntegerOverflow=on  InputSameDT=on
  MAPcor : Outport
  wires:
  MAP Estimate/1(map) -> Switch4/1
  In2/1 -> Bus Selector1/1
  Switch4/1 -> MAPcor/1
  In1/1 -> [sensors]
  [sensors] -> MAP Estimate/1(Sensors)
  [sensors] -> Bus Selector2/1
  Bus Selector2/1 -> Switch4/3  "<MAP>"
  Bus Selector1/1 -> MAP Estimate/Enable, Switch4/2  "<MAP_fail>"

== system mwrc04_fullvehicle/ECU/ECU Application Software/Sensor correction and  Fault Redundancy/Speed Accomodation ==
  sensors : Inport
  failures : Inport  Port=2
  Bus Selector1 : BusSelector  OutputSignals=Neng_fail
  Bus Selector2 : BusSelector  OutputSignals=Neng
  Speed Estimate : Subsystem
  Switch3 : Switch  Threshold=1  SaturateOnIntegerOverflow=on  InputSameDT=on
  Ncor : Outport
  wires:
  Speed Estimate/1(we) -> Switch3/1
  failures/1 -> Bus Selector1/1
  Switch3/1 -> Ncor/1
  sensors/1 -> [sensors]
  [sensors] -> Speed Estimate/1(Sensors)
  [sensors] -> Bus Selector2/1
  Bus Selector2/1 -> Switch3/3  "<Neng>"
  Bus Selector1/1 -> Speed Estimate/Enable, Switch3/2  "<Neng_fail>"

== system mwrc04_fullvehicle/ECU/ECU Application Software/Sensor correction and  Fault Redundancy/Throttle Accomodation ==
  sensors : Inport
  failures : Inport  Port=2
  Bus Selector1 : BusSelector  OutputSignals=throttle_fail
  Bus Selector2 : BusSelector  OutputSignals=throttle
  Switch : Switch  Threshold=1  SaturateOnIntegerOverflow=on  InputSameDT=on
  Throttle Estimate : Subsystem
  ThrottleCor : Outport
  wires:
  failures/1 -> Bus Selector1/1
  Throttle Estimate/1(throtle) -> Switch/1
  Switch/1 -> ThrottleCor/1
  Bus Selector2/1 -> Switch/3  "<throttle>"
  sensors/1 -> [sensors]
  [sensors] -> Throttle Estimate/1(Sensors)
  [sensors] -> Bus Selector2/1
  Bus Selector1/1 -> Switch/2, Throttle Estimate/Enable  "<throttle_fail>"

== system mwrc04_fullvehicle/ECU/ECU Application Software/Fuel  Calculation/Switchable Compensation/LOW Mode ==
  In1 : Inport
  Enable : EnablePort  StatesWhenEnabling=reset
  Discrete Transfer Fcn (with initial outputs) : simulink_extras/Additional Discrete/Discrete Transfer Fcn (with initial outputs)  N=num  D=den  U0=u0  Y0=y0  TS=Ts
  Out1 : Outport  InitialOutput=y0
  wires:
  Discrete Transfer Fcn (with initial outputs)/1 -> Out1/1
  In1/1 -> Discrete Transfer Fcn (with initial outputs)/1

== system mwrc04_fullvehicle/ECU/ECU Application Software/Fuel  Calculation/Switchable Compensation/RICH Mode ==
  In1 : Inport
  Enable : EnablePort  StatesWhenEnabling=reset
  Discrete Transfer Fcn (with initial outputs) : simulink_extras/Additional Discrete/Discrete Transfer Fcn (with initial outputs)  N=num  D=den  U0=u0  Y0=y0  TS=Ts
  Out1 : Outport  InitialOutput=y0
  wires:
  In1/1 -> Discrete Transfer Fcn (with initial outputs)/1
  Discrete Transfer Fcn (with initial outputs)/1 -> Out1/1

== system mwrc04_fullvehicle/ECU/ECU Application Software/Sensor correction and  Fault Redundancy/MAP Accomodation/MAP Estimate ==
  note: MAP Estimation
  Sensors : Inport
  Enable : EnablePort
  Bus Selector2 : BusSelector  OutputSignals=Neng,throttle
  Pressure Estimate (2-D) : Lookup2D  RowIndex=SpeedVect  ColumnIndex=ThrotVect  OutputValues=PressEst  SaturateOnIntegerOverflow=on  InputSameDT=on
  map : Outport  InitialOutput=0
  wires:
  Sensors/1 -> Bus Selector2/1
  Bus Selector2/1 -> Pressure Estimate (2-D)/1  "<Neng>"
  Bus Selector2/2 -> Pressure Estimate (2-D)/2  "<throttle>"
  Pressure Estimate (2-D)/1 -> map/1

== system mwrc04_fullvehicle/ECU/ECU Application Software/Sensor correction and  Fault Redundancy/Speed Accomodation/Speed Estimate ==
  note: Speed Estimation
  Sensors : Inport
  Enable : EnablePort
  Bus Selector2 : BusSelector  OutputSignals=throttle,MAP
  Speed Table (2-D) : Lookup2D  RowIndex=ThrotVect  ColumnIndex=press  OutputValues=SpeedEst  SaturateOnIntegerOverflow=on  InputSameDT=on
  we : Outport  InitialOutput=0
  wires:
  Speed Table (2-D)/1 -> we/1
  Sensors/1 -> Bus Selector2/1
  Bus Selector2/2 -> Speed Table (2-D)/2  "<MAP>"
  Bus Selector2/1 -> Speed Table (2-D)/1  "<throttle>"

== system mwrc04_fullvehicle/ECU/ECU Application Software/Sensor correction and  Fault Redundancy/Throttle Accomodation/Throttle Estimate ==
  note: Throttle Estimation
  Sensors : Inport
  Enable : EnablePort
  Bus Selector2 : BusSelector  OutputSignals=Neng,MAP
  Thrott Estimation Table (2-D) : Lookup2D  RowIndex=SpeedVect  ColumnIndex=press  OutputValues=ThrotEst  SaturateOnIntegerOverflow=on  InputSameDT=on
  throtle : Outport  InitialOutput=0
  wires:
  Bus Selector2/1 -> Thrott Estimation Table (2-D)/1  "<Neng>"
  Bus Selector2/2 -> Thrott Estimation Table (2-D)/2  "<MAP>"
  Thrott Estimation Table (2-D)/1 -> throtle/1
  Sensors/1 -> Bus Selector2/1

== stateflow chart ECU/ECU Application Software/Mode Logic/control logic ==
  settings: updateMethod=DISCRETE  sampleTime=0.01
  state Oxygen_Sensor_Mode [parallel]
    settings: description=This state determines the validity of the exhaust gas oxygen sensor (EGO) data.
    state O2_fail
      entry: fail_state[O2] = 1;
      settings: description=The EGO sensor has failed.
    state O2_warmup
      entry: fail_state[O2] = 1;
      settings: description=The EGO sensor must come up to temperature before its data is reliable.
    state O2_normal
      entry: fail_state[O2] = 0;
      settings: description=Normal EGO sensor operation gives a reliable indication of excess oxygen in the exhaust gas, from which air/fuel mixture can be inferred.
    O2_fail -> O2_normal : [Ego < max_ego] /
        | Sens_Failure_Counter.DEC
    O2_normal -> O2_fail : [Ego > max_ego]/
        | Sens_Failure_Counter.INC
      settings: description=The failure condition is indicated by excessive output voltage.
    (default) -> O2_warmup
    O2_warmup -> O2_normal : [t > o2_t_thresh]
      settings: description=It is assumed that the time o2_t_thresh is sufficient for the sensor to warm up to operational temperature.
  state Pressure_Sensor_Mode [parallel]
    settings: description=This state assesses the validity of the manifold absolute pressure (MAP) sensor.
    state press_norm
      entry:  fail_state[PRESS] = 0
      settings: description=The manifold pressure sensor gives a reliable indication of absolute pressure (MAP).
    state press_fail
      entry: fail_state[PRESS] = 1
      settings: description=The pressure sensor (manifold, or MAP) no longer produces reliable data.
    press_norm -> press_fail : [press > max_press | press < min_press]
        | /Sens_Failure_Counter.INC
    (default) -> press_norm
    press_fail -> press_norm : [press > min_press & press < max_press] /
        | Sens_Failure_Counter.DEC
  state Throttle_Sensor_Mode [parallel]
    settings: description=This state determines the validity of the throttle sensor signal.
    state throt_norm
      entry: fail_state[THROT] = 0;
      settings: description=The throttle sensor gives a reliable indication of the angle of the throttle plate.
    state throt_fail
      entry: fail_state[THROT] = 1;
      settings: description=Signal levels indicate that the throttle sensor data is no longer valid.
    throt_norm -> throt_fail : [throt> max_throt | throt < min_throt]/
        | Sens_Failure_Counter.INC
      settings: description=A failure is indicated by data which is outside the expected range, typically due to an open or short circuit.
    (default) -> throt_norm
    throt_fail -> throt_norm : [throt >  min_throt & throt < max_throt]
        | / Sens_Failure_Counter.DEC
  state Speed_Sensor_Mode [parallel]
    settings: description="This state infers the validity of the speed sensor data.  A failure is indicated by the presence of manifold vacuum at zero speed."
    state speed_norm
      entry: fail_state[SPEED] = 0
      settings: description=The speed sensor data accurately represents the engine speed.
    state speed_fail
      entry: fail_state[SPEED] = 1
      settings: description=The engine speed data is no longer available.
    speed_norm -> speed_fail : [speed==0 & press < zero_thresh]/
        | Sens_Failure_Counter.INC
      settings: description="Loss of a reliable speed sensor signal will indicate zero speed.  This is deemed invalid when the manifold vacuum indicates otherwise."
    (default) -> speed_norm
    speed_fail -> speed_norm : [speed > 0] /
        | Sens_Failure_Counter.DEC
  state Sens_Failure_Counter [parallel]
    settings: description=This state maintains a count of the number of sensors in failure mode.
    state MultiFail
      settings: description=This state represents any of the conditions in which more than one sensor is in failure mode.
      state FL3
        settings: description=Three of the engine sensors have failed.
      state FL4
        settings: description=All four of the engine sensors have failed.
      state FL2
        settings: description=Two of the engine sensors have failed.
      FL3 -> FL4 : INC
      FL2 -> FL3 : INC
      FL4 -> FL3 : DEC
      FL3 -> FL2 : DEC
    state FL1
      settings: description=One of the engine sensors has failed.
    state FL0
      settings: description=Zero failures; all sensors are operational.
    (default) -> FL0
    FL0 -> FL1 : INC
    FL1 -> FL2 : INC
    FL2 -> FL1 : DEC
    FL1 -> FL0 : DEC
  state Fueling_Mode [parallel]
    settings: description=This state interprets the other states in the chart to directly control the fueling mode.
    state Fuel_Disabled
      entry: fuel_mode = DISABLED
      settings: description=The fuel is completely shut off while in this state.
      state Overspeed
        settings: description=The speed is dangerously high, so shut off the fuel.
      state Shutdown
        settings: description=Cut off system operation due to multiple sensor failures.
      Overspeed -> (junction 35) : [in(speed_norm) & ...
          | speed < (max_speed - hys)]
      (junction 35) -> Shutdown : [in(MultiFail)]
    state Running
      settings: description=The fuel is actively controlled while in this state.
      (history)
      state Low_Emissions
        entry: fuel_mode = LOW
        (history)
        state Normal
          settings: description=All sensors are in correct operating modes, so effective closed-loop mixture control can be used.
        state Warmup
          settings: description="The sensors are all operational, but the oxygen (EGO) sensor is warming up.  We'll target a stoichiometric ratio, nonetheless, but won't close the loop around exhaust gas oxygen."
        (junction 36) -> Normal
        Warmup -> (junction 36) : [in(O2_normal)]
      state Rich_Mixture
        entry: fuel_mode = RICH
        settings: description=This mode enriches the mixture, lowering the air/fuel ratio.
        state Single_Failure
          settings: description=Continue uninterrupted engine operation, but with a richer mixture.
      Normal -> Single_Failure : [in(FL1)]
      Single_Failure -> Normal : [in(FL0)]
      (junction 36) -> Single_Failure : [in(FL1)]
    Running -> Overspeed : [ speed > max_speed ]
    (junction 35) -> Running : [!in(MultiFail)]
    Running -> Shutdown : enter(MultiFail)
    Shutdown -> Rich_Mixture : exit(MultiFail)
    (default) -> Warmup
  data: throt input double [0..120]; speed input double [0..1000]; Ego input double [0..2]; press input double [0..2]; fail_state output boolean size=4 [0..1]; fuel_mode output uint8 [1..3]; o2_t_thresh constant double [0..60]; max_ego constant double [0..2]; max_press constant double [0..2]; min_press constant double [0..2]; min_throt constant double [0..120]; max_throt constant double [0..120]; zero_thresh constant double [0..2]; max_speed constant double [0..1000]; hys constant double [0..1000]; LOW constant double; RICH constant double; DISABLED constant double; O2 constant uint8 =3; PRESS constant uint8 =4; THROT constant uint8 =1; SPEED constant uint8 =2
  data throt settings: units=degrees  description=throttle plate angle
  data speed settings: units=rad/sec  description=engine angular velocity
  data Ego settings: units=volts  description=Exhaust Gas Oxygen
  data press settings: units=bar (absolute)  description=Manifold Absolute Pressure (MAP)
  data fail_state settings: units=fail/ok  description=array of failure indications for use by Simulink model
  data fuel_mode settings: units=enumerated  description=fuel control mode: LOW = stoichiometric mixture, RICH = rich mixture, DISABLED = shut down
  data o2_t_thresh settings: units=sec  description=Time required to warm the EGO sensor sufficiently for valid data.
  data max_ego settings: units=volts  description=parameter represents the upper end of the EGO sensor range
  data max_press settings: units=bar (absolute)  description=parameter represents the upper limt of valid pressure readings
  data min_press settings: units=bar (absolute)  description=parameter for the lower end of the valid pressure sensor range
  data min_throt settings: units=degrees  description=minimum valid throttle angle
  data max_throt settings: units=degrees  description=parameter to indicate the maximum valid throttle angle reading
  data zero_thresh settings: units=bar (absolute)  description=minimum manifold pressure expected at zero speed
  data max_speed settings: units=rad/sec  description=parameter for the upper end of the safe engine speed range
  data hys settings: units=rad/sec  description=Hysteresis in the upper speed limit to avoid chatter at the threshold.
  data LOW settings: description="constant represents \"low emissions\" or stoichiometric fuel mixture mode"
  data RICH settings: description=constant represents rich fuel mixture mode
  data DISABLED settings: description=constant represents zero fuel mode
  data O2 settings: units=index  description=index into fail_state
  data PRESS settings: units=index  description=index into fail_state
  data THROT settings: units=index  description=index into fail_state
  data SPEED settings: units=index
  events: DEC local EITHER_EDGE_EVENT; INC local EITHER_EDGE_EVENT

== stateflow chart TCU/shift_logic ==
  settings: updateMethod=DISCRETE  sampleTime=0.04
  state gear_state [parallel]
    state fourth
      entry: gear = 4;
    state second
      entry: gear = 2;
    state third
      entry: gear = 3;
    state first
      entry: gear = 1;
    third -> fourth : UP
    second -> third : UP
    first -> second : UP
    (default) -> first
    fourth -> third : DOWN
    third -> second : DOWN
    second -> first : DOWN
  state selection_state [parallel]
    during: CALC_TH;
    state downshifting
    state upshifting
    state steady_state
    (default) -> steady_state
    steady_state -> upshifting : [speed > up_th]
    steady_state -> downshifting : [speed < down_th]
    upshifting -> steady_state : [speed < up_th]
    downshifting -> steady_state : [speed > down_th]
    downshifting -> steady_state : after(TWAIT,tick)
        | [speed <= down_th]
        | {gear_state.DOWN}
    upshifting -> steady_state : after(TWAIT,tick)
        | [speed >= up_th]
        | {gear_state.UP}
  data: speed input double; gear output uint8 [1..4]; TWAIT constant uint8; up_th input double; down_th input double
  data speed settings: units=double
  data gear settings: units=int
  events: DOWN local EITHER_EDGE_EVENT; UP local EITHER_EDGE_EVENT; CALC_TH output FUNCTION_CALL_EVENT
